simulink model "TV_2021"  (R2017b)
settings: Solver=VariableStepAuto  StartTime=0.0  StopTime=10.0  RelTol=1e-3
undefined symbols (not defined in the file): sigbuilder_block
libraries: simulink x6
(part 1 of 13)
settings Model: Creator=Eric  LastModifiedBy=GERARD
settings DataIOCC: ReturnWorkspaceOutputs=on
settings SFSimCC: SimUseLocalCustomCode=on
settings RTWCC: RTWUseLocalCustomCode=on

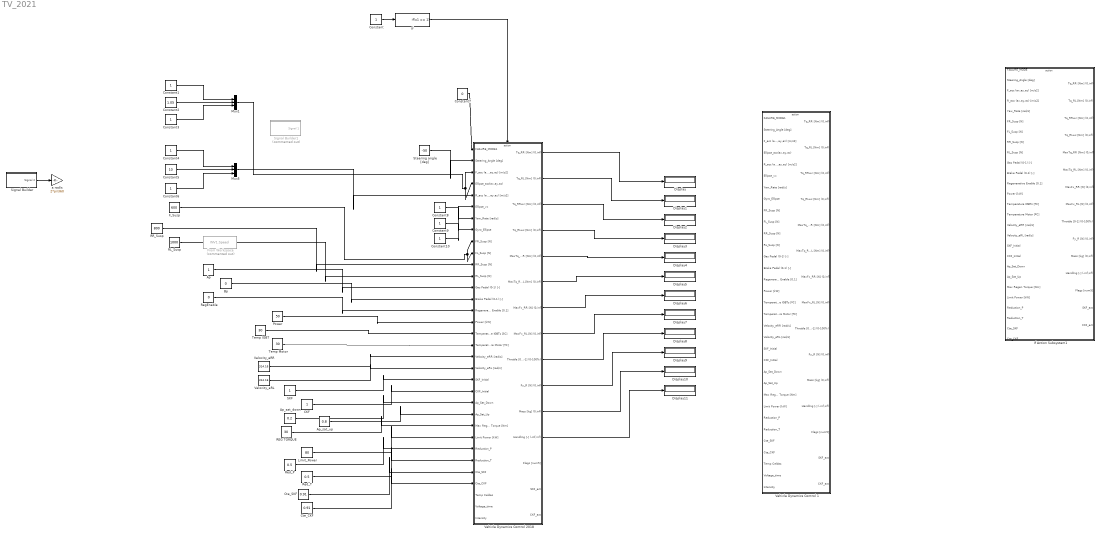
== system TV_2021 ==
  Ap : Constant
  Ap_sat_down : Constant  Value=0.2
  Ap_sat_up : Constant  Value=0.8
  Bp : Constant  Value=0
  CKF : Constant
  Constant{,1,3..4,6,8..10} (8 alike) : Constant
  Constant2 : Constant  Value=1.05
  Constant5 : Constant  Value=10
  Constant7 : Constant  Value=0
  Cte_CKF : Constant  Value=0.91
  Cte_SKF : Constant  Value=0.91
  Display{,1..11} (12 alike) : Display
  F_Susp : Constant  Value=600
  From Workspace : FromWorkspace  Commented=on  VariableName=INV1.Speed  SampleTime=0.05  OutputAfterFinalValue=Holding final value
  If : If  IfExpression=u1 == 1  ShowElse=off
  If Action Subsystem1 : Subsystem  TreatAsAtomicUnit=on
  Limit_Power : Constant  Value=80
  Mux1 : Mux  Inputs=3
  Mux5 : Mux  Inputs=3
  Power : Constant  Value=50
  REG TORQUE : Constant  Value=30
  RL_Susp : Constant  Value=1000
  RR_Susp : Constant  Value=800
  Red_P : Constant  Value=0.5
  Red_T : Constant  Value=0.5
  RegEnable : Constant  Value=0
  SKF : Constant
  Signal Builder : Subsystem  Tag=STV Subsys  LoadFcn=sigbuilder_block('load');  StartFcn=sigbuilder_block('start');  StopFcn=sigbuilder_block('stop');  ClipboardFcn=sigbuilder_block('clipboard');  mask(Sigbuilder block){tuvar=[0:10]}
      mask help: Simulink:masks:SigbuilderBlock_MD
      mask init:
      | if ~strcmp(get_param(bdroot(gcbh),'SimulationStatus'),'stopped') tuvar = sigbuilder_block('maskInit'); end
      settings: CopyFcn=sigbuilder_block('copy');  DeleteFcn=sigbuilder_block('delete');  ModelCloseFcn=sigbuilder_block('modelClose');  PreSaveFcn=sigbuilder_block('preSave');  PauseFcn=sigbuilder_block('pause');  ContinueFcn=sigbuilder_block('continue');  NameChangeFcn=sigbuilder_block('namechange');  OpenFcn=sigbuilder_block('open',[5.4 33 1141.2 514.8 ]);  CloseFcn=sigbuilder_block('close');
      mask Display: plot(0, 0, 100, 100,[2, 2, 32, 32, 2], [68, 8, 8, 68, 68],[32, 2], [38, 38], [32, 19, 2],[53, 60, 44], [32, 17, 17, 2],[16, 16, 31, 31]);txt = getActiveGroup(gcbh);text(2, 100, txt,'verticalAlignment', 'top');
  Signal Builder1 : Subsystem  Tag=STV Subsys  Commented=on  LoadFcn=sigbuilder_block('load');  StartFcn=sigbuilder_block('start');  StopFcn=sigbuilder_block('stop');  ClipboardFcn=sigbuilder_block('clipboard');  mask(Sigbuilder block){tuvar=[0:10]}
      mask help: Simulink:masks:SigbuilderBlock_MD
      mask init:
      | if ~strcmp(get_param(bdroot(gcbh),'SimulationStatus'),'stopped') tuvar = sigbuilder_block('maskInit'); end
      settings: CopyFcn=sigbuilder_block('copy');  DeleteFcn=sigbuilder_block('delete');  ModelCloseFcn=sigbuilder_block('modelClose');  PreSaveFcn=sigbuilder_block('preSave');  PauseFcn=sigbuilder_block('pause');  ContinueFcn=sigbuilder_block('continue');  NameChangeFcn=sigbuilder_block('namechange');  OpenFcn=sigbuilder_block('open',[5.4 33 1141.2 516.6 ]);  CloseFcn=sigbuilder_block('close');
      mask Display: plot(0, 0, 100, 100,[2, 2, 32, 32, 2], [68, 8, 8, 68, 68],[32, 2], [38, 38], [32, 19, 2],[53, 60, 44], [32, 17, 17, 2],[16, 16, 31, 31]);txt = getActiveGroup(gcbh);text(2, 100, txt,'verticalAlignment', 'top');
  Steering angle [deg] : Constant  Value=-50
  Temp IGBT : Constant  Value=30
  Temp Motor : Constant  Value=30
  Vehicle Dynamics Control 1 : Subsystem
  Vehicle Dynamics Control 2018 : Subsystem
  Velocity_eRL : Constant  Value=314.16
  Velocity_eRR : Constant  Value=314.16
  a rad/s : Gain  Gain=2*pi/360
  wires:
  If/1 -> Vehicle Dynamics Control 2018/Action
  Constant/1 -> If/1
  Vehicle Dynamics Control 2018/1(Tq_RR [Nm] (0,inf)) -> Display/1
  Vehicle Dynamics Control 2018/2(Tq_RL [Nm] (0,inf)) -> Display1/1
  Vehicle Dynamics Control 2018/3(Tq_RRwc [Nm] (0,inf)) -> Display2/1
  Vehicle Dynamics Control 2018/4(Tq_RLwc [Nm] (0,inf)) -> Display3/1
  Vehicle Dynamics Control 2018/5(MaxTq_RR [Nm] (0,inf)) -> Display4/1
  Vehicle Dynamics Control 2018/6(MaxTq_RL [Nm] (0,inf)) -> Display5/1
  Vehicle Dynamics Control 2018/7(MaxFx_RR [N] (0,inf)) -> Display6/1
  Vehicle Dynamics Control 2018/8(MaxFx_RL [N] (0,inf)) -> Display7/1
  Vehicle Dynamics Control 2018/9(Throttle [0-1] (0-100%)) -> Display8/1
  Vehicle Dynamics Control 2018/10(Fy_R [N] (0,inf)) -> Display9/1
  Vehicle Dynamics Control 2018/11(Mass [kg] (0,inf)) -> Display10/1
  Vehicle Dynamics Control 2018/12(Handling [-] (-inf,inf)) -> Display11/1
  Bp/1 -> Vehicle Dynamics Control 2018/14(Brake Pedal (0-1) [-])
  RegEnable/1 -> Vehicle Dynamics Control 2018/15(Regenerative Enable [0,1])
  Red_T/1 -> Vehicle Dynamics Control 2018/28(Reduction_T)
  Cte_CKF/1 -> Vehicle Dynamics Control 2018/30(Cte_CKF)
  Red_P/1 -> Vehicle Dynamics Control 2018/27(Reduction_P)
  Constant5/1 -> Mux5/2
  Constant1/1 -> Mux1/1
  Mux1/1 -> Vehicle Dynamics Control 2018/4(Ellipse_acc(ax,ay,az)), Vehicle Dynamics Control 2018/3(F_acc (ax,ay,az) [m/s2])
  Mux5/1 -> Vehicle Dynamics Control 2018/5(R_acc (ax,ay,az) [m/s2])
  Constant6/1 -> Mux5/3
  Constant3/1 -> Mux1/3
  Velocity_eRR/1 -> Vehicle Dynamics Control 2018/19(Velocity_eRR [rad/s])
  RL_Susp/1 -> Vehicle Dynamics Control 2018/12(RL_Susp [N])
  Constant4/1 -> Mux5/1
  Cte_SKF/1 -> Vehicle Dynamics Control 2018/29(Cte_SKF)
  SKF/1 -> Vehicle Dynamics Control 2018/21(SKF_Initial)
  Velocity_eRL/1 -> Vehicle Dynamics Control 2018/20(Velocity_eRL [rad/s])
  Limit_Power/1 -> Vehicle Dynamics Control 2018/26(Limit Power [kW])
  F_Susp/1 -> Vehicle Dynamics Control 2018/9(FR_Susp [N]), Vehicle Dynamics Control 2018/10(FL_Susp [N])
  Ap/1 -> Vehicle Dynamics Control 2018/13(Gas Pedal (0-1) [-])
  CKF/1 -> Vehicle Dynamics Control 2018/22(CKF_Initial)
  Signal Builder/1(Signal 2) -> a rad/s/1
  Steering angle [deg]/1 -> Vehicle Dynamics Control 2018/2(Steering_Angle [deg])
  Constant2/1 -> Mux1/2
  Constant7/1 -> Vehicle Dynamics Control 2018/1(FAILURE_MODE1)
  REG TORQUE/1 -> Vehicle Dynamics Control 2018/25(Max Regen Torque [Nm])
  Ap_sat_up/1 -> Vehicle Dynamics Control 2018/24(Ap_Sat_Up)
  Ap_sat_down/1 -> Vehicle Dynamics Control 2018/23(Ap_Sat_Down)
  Temp Motor/1 -> Vehicle Dynamics Control 2018/18(Temperature Motor [ºC])
  Temp IGBT/1 -> Vehicle Dynamics Control 2018/17(Temperature IGBTs [ºC])
  Power/1 -> Vehicle Dynamics Control 2018/16(Power [kW])
  RR_Susp/1 -> Vehicle Dynamics Control 2018/11(RR_Susp [N])
  Constant8/1 -> Vehicle Dynamics Control 2018/6(Ellipse_vx)
  Constant9/1 -> Vehicle Dynamics Control 2018/7(Yaw_Rate [rad/s])
  Constant10/1 -> Vehicle Dynamics Control 2018/8(Gyro_Ellipse)

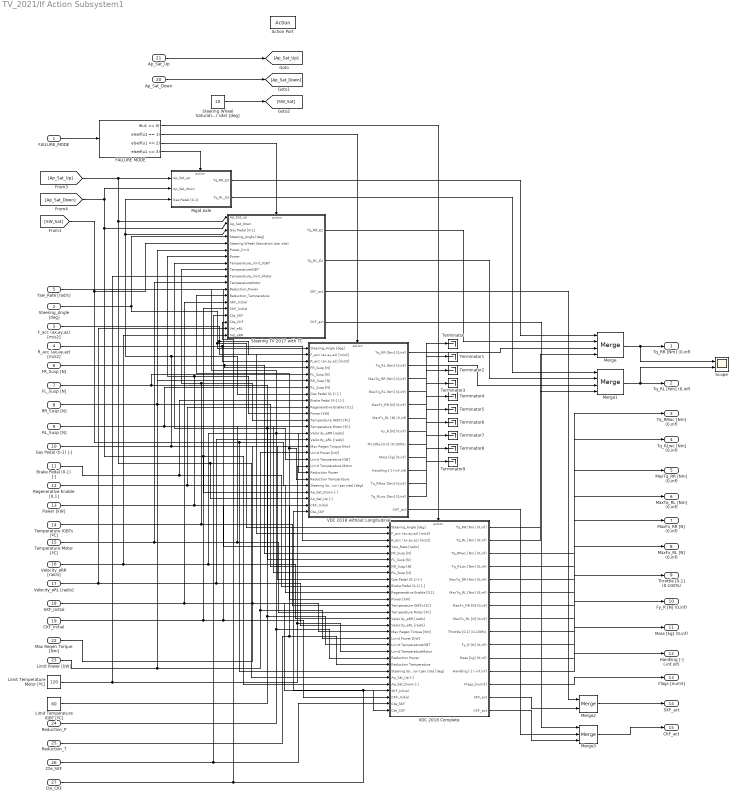
== system TV_2021/If Action Subsystem1 ==
  FAILURE_MODE : Inport
  Steering_Angle [deg] : Inport  Port=2
  F_acc (ax,ay,az) [m/s2] : Inport  Port=3
  R_acc (ax,ay,az) [m/s2] : Inport  Port=4
  Yaw_Rate [rad/s] : Inport  Port=5
  FR_Susp [N] : Inport  Port=6
  FL_Susp [N] : Inport  Port=7
  RR_Susp [N] : Inport  Port=8
  RL_Susp [N] : Inport  Port=9
  Gas Pedal (0-1) [-] : Inport  Port=10
  Brake Pedal (0-1) [-] : Inport  Port=11
  Regenerative Enable [0,1] : Inport  Port=12
  Power [kW] : Inport  Port=13
  Temperature IGBTs [ºC] : Inport  Port=14
  Temperature Motor [ºC] : Inport  Port=15
  Velocity_eRR [rad/s] : Inport  Port=16
  Velocity_eRL [rad/s] : Inport  Port=17
  SKF_Initial : Inport  Port=18
  CKF_Initial : Inport  Port=19
  Ap_Sat_Down : Inport  Port=20
  Ap_Sat_Up : Inport  Port=21
  Max Regen Torque [Nm] : Inport  Port=22
  Limit Power [kW] : Inport  Port=23
  Reduction_P : Inport  Port=24
  Reduction_T : Inport  Port=25
  Cte_SKF : Inport  Port=26
  Cte_CKF : Inport  Port=27
  Action Port : ActionPort
  FAILURE MODE : If  IfExpression=u1 == 0  ElseIfExpressions=u1 == 1, u1 == 2, u1 == 3  ShowElse=off
  Limit Temperature IGBT [ºC] : Constant  Value=60
  Limit Temperature Motor [ºC] : Constant  Value=120
  Merge : Merge  Inputs=4
  Merge1 : Merge  Inputs=4
  Merge2 : Merge
  Merge3 : Merge  Inputs=3
  Rigid Axle : Subsystem  TreatAsAtomicUnit=on
  Scope : Scope  NumInputPorts=2
  Steering TV 2017 with TC : Subsystem  TreatAsAtomicUnit=on
  "Steering Wheel Saturation (per site) [deg] " : Constant  Value=10
  Terminator{,1..9} (10 alike) : Terminator
  VDC 2018 Complete : Subsystem  TreatAsAtomicUnit=on
  VDC 2018 without Longitudinal : Subsystem  TreatAsAtomicUnit=on
  Tq_RR [Nm] (0,inf) : Outport
  Tq_RL [Nm] (0,inf) : Outport  Port=2
  Tq_RRwc [Nm] (0,inf) : Outport  Port=3
  Tq_RLwc [Nm] (0,inf) : Outport  Port=4
  MaxTq_RR [Nm] (0,inf) : Outport  Port=5
  MaxTq_RL [Nm] (0,inf) : Outport  Port=6
  MaxFx_RR [N] (0,inf) : Outport  Port=7
  MaxFx_RL [N] (0,inf) : Outport  Port=8
  Throttle [0-1] (0-100%) : Outport  Port=9
  Fy_R [N] (0,inf) : Outport  Port=10
  Mass [kg] (0,inf) : Outport  Port=11
  Handling [-] (-inf,inf) : Outport  Port=12
  Flags [num5] : Outport  Port=13
  SKF_act : Outport  Port=14
  CKF_act : Outport  Port=15
  wires:
  RL_Susp [N]/1 -> VDC 2018 Complete/8(RL_Susp [N]), VDC 2018 without Longitudinal/7(RL_Susp [N])
  R_acc (ax,ay,az) [m/s2]/1 -> VDC 2018 Complete/3(R_acc (ax,ay,az) [m/s2]), VDC 2018 without Longitudinal/3(R_acc (ax,ay,az) [m/s2])
  Steering TV 2017 with TC/4(CKF_act) -> Merge3/1
  Cte_SKF/1 -> Steering TV 2017 with TC/16(Cte_SKF), VDC 2018 Complete/28(Cte_SKF)
  VDC 2018 without Longitudinal/13(CKF_act) -> Merge3/2
  Steering TV 2017 with TC/3(SKF_act) -> Merge2/1
  Merge3/1 -> CKF_act/1
  VDC 2018 Complete/10(Fy_R [N] (0,inf)) -> Fy_R [N] (0,inf)/1
  Yaw_Rate [rad/s]/1 -> VDC 2018 Complete/4(Yaw_Rate [rad/s])
  VDC 2018 without Longitudinal/2(Tq_RL [Nm] (0,inf)) -> Merge1/3
  Merge2/1 -> SKF_act/1
  VDC 2018 Complete/15(CKF_act) -> Merge3/3
  VDC 2018 without Longitudinal/12(Tq_RLwc [Nm] (0,inf)) -> Terminator9/1
  VDC 2018 without Longitudinal/9(Mass [kg] (0,inf)) -> Terminator6/1
  Gas Pedal (0-1) [-]/1 -> VDC 2018 Complete/9(Gas Pedal (0-1) [-]), Steering TV 2017 with TC/3(Gas Pedal [0-1]), Rigid Axle/3(Gas Pedal [0-1]), VDC 2018 without Longitudinal/8(Gas Pedal (0-1) [-])
  Limit Temperature IGBT [ºC]/1 -> VDC 2018 without Longitudinal/18(Limit Temperature IGBT), Steering TV 2017 with TC/8(Temperature_limit_IGBT), VDC 2018 Complete/19(Limit TemperatureIGBT)
  SKF_Initial/1 -> VDC 2018 Complete/26(SKF_Initial), Steering TV 2017 with TC/14(SKF_Initial)
  Cte_CKF/1 -> Steering TV 2017 with TC/17(Cte_CKF), VDC 2018 without Longitudinal/26(Cte_CKF), VDC 2018 Complete/29(Cte_CKF)
  VDC 2018 Complete/13(Flags_[num5]) -> Flags [num5]/1
  VDC 2018 without Longitudinal/4(MaxTq_RL [Nm] (0,inf)) -> Terminator1/1
  VDC 2018 without Longitudinal/11(Tq_RRwc [Nm] (0,inf)) -> Terminator8/1
  Steering_Angle [deg]/1 -> VDC 2018 Complete/1(Steering_Angle [deg]), VDC 2018 without Longitudinal/1(Steering_Angle [deg]), Steering TV 2017 with TC/4(Steering_Angle [deg])
  Reduction_P/1 -> Steering TV 2017 with TC/12(Reduction_Power), VDC 2018 without Longitudinal/20(Reduction Power), VDC 2018 Complete/21(Reduction Power)
  VDC 2018 without Longitudinal/3(MaxTq_RR [Nm] (0,inf)) -> Terminator/1
  Brake Pedal (0-1) [-]/1 -> VDC 2018 Complete/10(Brake Pedal (0-1) [-]), VDC 2018 without Longitudinal/9(Brake Pedal (0-1) [-])
  VDC 2018 without Longitudinal/6(MaxFx_RL [N] (0,inf)) -> Terminator3/1
  VDC 2018 Complete/11(Mass [kg] (0,inf)) -> Mass [kg] (0,inf)/1
  Velocity_eRR [rad/s]/1 -> Steering TV 2017 with TC/19(Vel_eRR), VDC 2018 without Longitudinal/14(Velocity_eRR [rad/s]), VDC 2018 Complete/15(Velocity_eRR [rad/s])
  VDC 2018 without Longitudinal/8(Throttle [0-1] (0-100%)) -> Terminator5/1
  F_acc (ax,ay,az) [m/s2]/1 -> VDC 2018 Complete/2(F_acc (ax,ay,az) [m/s2]), VDC 2018 without Longitudinal/2(F_acc (ax,ay,az) [m/s2])
  VDC 2018 without Longitudinal/7(Fy_R [N] (0,inf)) -> Terminator4/1
  Ap_Sat_Up/1 -> [Ap_Sat_Up]
  Merge/1 -> Scope/1, Tq_RR [Nm] (0,inf)/1
  VDC 2018 Complete/12(Handling [-] (-inf,inf)) -> Handling [-] (-inf,inf)/1
  VDC 2018 without Longitudinal/1(Tq_RR [Nm] (0,inf)) -> Merge/3
  Max Regen Torque [Nm]/1 -> VDC 2018 without Longitudinal/16(Max Regen Torque [Nm]), VDC 2018 Complete/17(Max Regen Torque [Nm])
  FR_Susp [N]/1 -> VDC 2018 without Longitudinal/4(FR_Susp [N]), VDC 2018 Complete/5(FR_Susp [N])
  VDC 2018 Complete/4(Tq_RLwc [Nm] (0,inf)) -> Tq_RLwc [Nm] (0,inf)/1
  VDC 2018 without Longitudinal/5(MaxFx_RR [N] (0,inf)) -> Terminator2/1
  VDC 2018 Complete/3(Tq_RRwc [Nm] (0,inf)) -> Tq_RRwc [Nm] (0,inf)/1
  Limit Temperature Motor [ºC]/1 -> VDC 2018 without Longitudinal/19(Limit Temperature Motor), VDC 2018 Complete/20(Limit TemperatureMotor), Steering TV 2017 with TC/10(Temperature_limit_Motor)
  Rigid Axle/2(Tq_RL_E3) -> Merge1/1
  VDC 2018 Complete/9(Throttle [0-1] (0-100%)) -> Throttle [0-1] (0-100%)/1
  Reduction_T/1 -> Steering TV 2017 with TC/13(Reduction_Temperature), VDC 2018 without Longitudinal/21(Reduction Temperature), VDC 2018 Complete/22(Reduction Temperature)
  [Ap_Sat_Up] -> Rigid Axle/1("Ap_Sat_up "), VDC 2018 Complete/24(Ap_Sat_Up [-]), VDC 2018 without Longitudinal/24(Ap_Sat_Up [-]), Steering TV 2017 with TC/1("Ap_Sat_up ")
  Temperature Motor [ºC]/1 -> VDC 2018 without Longitudinal/13(Temperature Motor [ºC]), VDC 2018 Complete/14(Temperature Motor [ºC]), Steering TV 2017 with TC/11(TemperatureMotor)
  VDC 2018 Complete/6(MaxTq_RL [Nm] (0,inf)) -> MaxTq_RL [Nm] (0,inf)/1
  CKF_Initial/1 -> Steering TV 2017 with TC/15(CKF_Initial), VDC 2018 without Longitudinal/25(CKF_Initial), VDC 2018 Complete/27(CKF_Initial)
  Velocity_eRL [rad/s]/1 -> Steering TV 2017 with TC/18(Vel_eRL), VDC 2018 without Longitudinal/15(Velocity_eRL [rad/s]), VDC 2018 Complete/16(Velocity_eRL [rad/s])
  VDC 2018 Complete/7(MaxFx_RR [N] (0,inf)) -> MaxFx_RR [N] (0,inf)/1
  VDC 2018 Complete/5(MaxTq_RR [Nm] (0,inf)) -> MaxTq_RR [Nm] (0,inf)/1
  VDC 2018 Complete/1(Tq_RR [Nm] (0,inf)) -> Merge/4
  Power [kW]/1 -> Steering TV 2017 with TC/7(Power), VDC 2018 without Longitudinal/11(Power [kW]), VDC 2018 Complete/12(Power [kW])
  VDC 2018 Complete/2(Tq_RL [Nm] (0,inf)) -> Merge1/4
  RR_Susp [N]/1 -> VDC 2018 without Longitudinal/6(RR_Susp [N]), VDC 2018 Complete/7(RR_Susp [N])
  VDC 2018 without Longitudinal/10(Handling [-] (-inf,inf)) -> Terminator7/1
  [SW_Sat] -> Steering TV 2017 with TC/5("Steering Wheel Saturation (per site) "), VDC 2018 Complete/23(Steering Saturation (per site) [deg]), VDC 2018 without Longitudinal/22(Steering Saturation (per site) [deg])
  Regenerative Enable [0,1]/1 -> VDC 2018 Complete/11(Regenerative Enable [0,1]), VDC 2018 without Longitudinal/10(Regenerative Enable [0,1])
  Limit Power [kW]/1 -> Steering TV 2017 with TC/6(Power_limit), VDC 2018 without Longitudinal/17(Limit Power [kW]), VDC 2018 Complete/18(Limit Power [kW])
  FAILURE MODE/3 -> Steering TV 2017 with TC/Action
  VDC 2018 Complete/14(SKF_act) -> Merge2/2
  [Ap_Sat_Down] -> VDC 2018 Complete/25(Ap_Sat_Down [-]), VDC 2018 without Longitudinal/23(Ap_Sat_Down [-]), Steering TV 2017 with TC/2(Ap_Sat_down), Rigid Axle/2(Ap_Sat_down)
  Steering TV 2017 with TC/2(Tq_RL_E2) -> Merge1/2
  Temperature IGBTs [ºC]/1 -> VDC 2018 Complete/13(Temperature IGBTs [ºC]), Steering TV 2017 with TC/9(TemperatureIGBT), VDC 2018 without Longitudinal/12(Temperature IGBTs [ºC])
  "Steering Wheel Saturation (per site) [deg] "/1 -> [SW_Sat]
  VDC 2018 Complete/8(MaxFx_RL [N] (0,inf)) -> MaxFx_RL [N] (0,inf)/1
  FL_Susp [N]/1 -> VDC 2018 without Longitudinal/5(FL_Susp [N]), VDC 2018 Complete/6(FL_Susp [N])
  Ap_Sat_Down/1 -> [Ap_Sat_Down]
  Merge1/1 -> Scope/2, Tq_RL [Nm] (0,inf)/1
  FAILURE MODE/4 -> Rigid Axle/Action
  Rigid Axle/1(Tq_RR_E3) -> Merge/1
  Steering TV 2017 with TC/1(Tq_RR_E2) -> Merge/2
  FAILURE_MODE/1 -> FAILURE MODE/1
  FAILURE MODE/1 -> VDC 2018 Complete/Action
  FAILURE MODE/2 -> VDC 2018 without Longitudinal/Action

== system TV_2021/Signal Builder ==
  Demux : Demux  Tag=STV Demux  Outputs=1
  FromWs : FromWorkspace  Tag=STV FromWs  VariableName=tuvar  SampleTime=0
      SigBuilderData=|
      | common.afterFinalStr = 'Extrapolate'
      | common.sampleTime = 0
      | dataSet.timeRange = [0 50]
      | dataSet.name = 'Group 1'
      | sbobj.Groups.Name = 'Group 1'
      | sbobj.Groups.Signals.Name = 'Signal 2'
      | sbobj.Groups.Signals.XData = [0 50]
      | sbobj.Groups.Signals.YData = [0 -150]
      | sbobj.Groups.TimeRange = [0 50]
  Signal 2 : Outport  Tag=STV Outport
  wires:
  FromWs/1 -> Demux/1
  Demux/1 -> Signal 2/1

== system TV_2021/Signal Builder1 ==
  Demux : Demux  Tag=STV Demux  Outputs=1
  FromWs : FromWorkspace  Tag=STV FromWs  VariableName=tuvar  SampleTime=0
      SigBuilderData=|
      | common.afterFinalStr = 'Extrapolate'
      | common.sampleTime = 0
      | dataSet.timeRange = [0 50]
      | dataSet.name = 'Group 1'
      | sbobj.Groups.Name = 'Group 1'
      | sbobj.Groups.Signals.Name = 'Signal 1'
      | sbobj.Groups.Signals.XData = [0 30 30 50]
      | sbobj.Groups.Signals.YData = [20 20 30 30]
      | sbobj.Groups.TimeRange = [0 50]
  Signal 1 : Outport  Tag=STV Outport
  wires:
  FromWs/1 -> Demux/1
  Demux/1 -> Signal 1/1

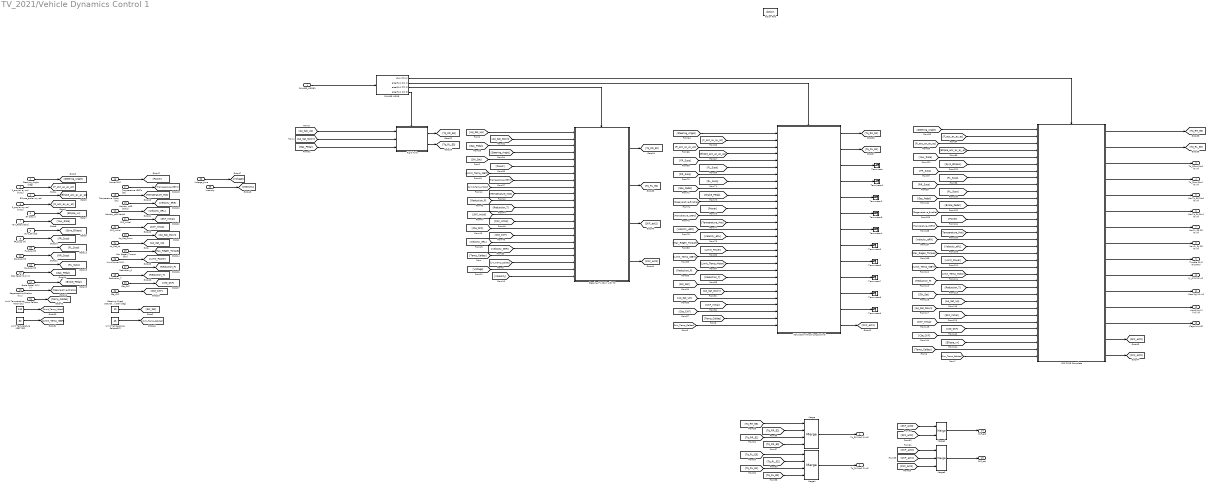
== system TV_2021/Vehicle Dynamics Control 1 ==
  FAILURE_MODE1 : Inport
  Steering_Angle [deg] : Inport  Port=2
  F_acc (ax,ay,az) [m/s2] : Inport  Port=3
  Ellipse_acc(ax,ay,az) : Inport  Port=4
  R_acc (ax,ay,az) [m/s2] : Inport  Port=5
  Ellipse_vx : Inport  Port=6
  Yaw_Rate [rad/s] : Inport  Port=7
  Gyro_Ellipse : Inport  Port=8
  FR_Susp [N] : Inport  Port=9
  FL_Susp [N] : Inport  Port=10
  RR_Susp [N] : Inport  Port=11
  RL_Susp [N] : Inport  Port=12
  Gas Pedal (0-1) [-] : Inport  Port=13
  Brake Pedal (0-1) [-] : Inport  Port=14
  Regenerative Enable [0,1] : Inport  Port=15
  Power [kW] : Inport  Port=16
  Temperature IGBTs [ºC] : Inport  Port=17
  Temperature Motor [ºC] : Inport  Port=18
  Velocity_eRR [rad/s] : Inport  Port=19
  Velocity_eRL [rad/s] : Inport  Port=20
  SKF_Initial : Inport  Port=21
  CKF_Initial : Inport  Port=22
  Ap_Sat_Down : Inport  Port=23
  Ap_Sat_Up : Inport  Port=24
  Max Regen Torque [Nm] : Inport  Port=25
  Limit Power [kW] : Inport  Port=26
  Reduction_P : Inport  Port=27
  Reduction_T : Inport  Port=28
  Cte_SKF : Inport  Port=29
  Cte_CKF : Inport  Port=30
  Temp Celdas : Inport  Port=31
  Voltage_time : Inport  Port=32
  Intensity : Inport  Port=33
  Action Port : ActionPort
  FAILURE MODE : If  IfExpression=u1 == 0  ElseIfExpressions=u1 == 1, u1 == 2, u1 == 3  ShowElse=off
  Limit Temperature Celdas[ºC] : Constant  Value=45
  Limit Temperature IGBT [ºC] : Constant  Value=60
  Limit Temperature Motor [ºC] : Constant  Value=110
  Merge : Merge  Inputs=4
  Merge1 : Merge  Inputs=4
  Merge2 : Merge
  Merge3 : Merge  Inputs=3
  Rigid Axle : Subsystem  TreatAsAtomicUnit=on
  Steering TV 2017 with TC : Subsystem  TreatAsAtomicUnit=on
  "Steering Wheel Saturation (per site) [deg] " : Constant  Value=10
  Terminator{,1..9} (10 alike) : Terminator
  VDC 2018 Complete : Subsystem  TreatAsAtomicUnit=on
  VDC 2018 without Longitudinal : Subsystem  TreatAsAtomicUnit=on
  Tq_RR [Nm] (0,inf) : Outport
  Tq_RL [Nm] (0,inf) : Outport  Port=2
  Tq_RRwc [Nm] (0,inf) : Outport  Port=3
  Tq_RLwc [Nm] (0,inf) : Outport  Port=4
  MaxTq_RR [Nm] (0,inf) : Outport  Port=5
  MaxTq_RL [Nm] (0,inf) : Outport  Port=6
  MaxFx_RR [N] (0,inf) : Outport  Port=7
  MaxFx_RL [N] (0,inf) : Outport  Port=8
  Throttle [0-1] (0-100%) : Outport  Port=9
  Fy_R [N] (0,inf) : Outport  Port=10
  Mass [kg] (0,inf) : Outport  Port=11
  Handling [-] (-inf,inf) : Outport  Port=12
  Flags [num5] : Outport  Port=13
  SKF_act : Outport  Port=14
  CKF_act : Outport  Port=15
  wires:
  [Intensity] -> Steering TV 2017 with TC/22(Corriente)
  [Voltage] -> Steering TV 2017 with TC/21(Voltage)
  Intensity/1 -> [Intensity]
  Voltage_time/1 -> [Voltage]
  [Lim_Temp_Celdas] -> VDC 2018 Complete/34(Limit_Temp_Celdas)
  [Temp_Celdas] -> VDC 2018 Complete/33(Temp_Celdas)
  [Lim_Temp_Celdas] -> VDC 2018 without Longitudinal/29(Lim_Temp_Celdas)
  [Temp_Celdas] -> VDC 2018 without Longitudinal/28(Temp_Celdas)
  [Lim_Temp_Celdas] -> Steering TV 2017 with TC/20(Lim_Temp_Celdas)
  [Temp_Celdas] -> Steering TV 2017 with TC/19(Temp_Celdas)
  Limit Temperature Celdas[ºC]/1 -> [Lim_Temp_Celdas]
  Temp Celdas/1 -> [Temp_Celdas]
  FAILURE MODE/4 -> Rigid Axle/Action
  FAILURE MODE/3 -> Steering TV 2017 with TC/Action
  FAILURE MODE/2 -> VDC 2018 without Longitudinal/Action
  FAILURE_MODE1/1 -> FAILURE MODE/1
  FAILURE MODE/1 -> VDC 2018 Complete/Action
  [Ellipse_vx] -> VDC 2018 Complete/32(Ellipse_vx)
  [SKF_Initial] -> VDC 2018 Complete/28(SKF_Initial)
  [Cte_SKF] -> VDC 2018 Complete/30(Cte_SKF)
  [Cte_CKF] -> VDC 2018 Complete/31(Cte_CKF)
  [Gyro_Ellipse] -> VDC 2018 Complete/6(Gyro_Ellipse)
  [Yaw_Rate] -> VDC 2018 Complete/5(Yaw_Rate [rad/s])
  [CKF_Initial] -> VDC 2018 Complete/29(CKF_Initial)
  [Ap_Sat_Up] -> VDC 2018 Complete/26(Ap_Sat_Up [-])
  [Ap_Sat_Down] -> VDC 2018 Complete/27(Ap_Sat_Down [-])
  [SW_Sat] -> VDC 2018 Complete/25(Steering Saturation (per site) [deg])
  [Reduction_T] -> VDC 2018 Complete/24(Reduction Temperature)
  [Reduction_P] -> VDC 2018 Complete/23(Reduction Power)
  [Limit_Temp_Motor] -> VDC 2018 Complete/22(Limit TemperatureMotor)
  [Limit_Temp_IGBT] -> VDC 2018 Complete/21(Limit TemperatureIGBT)
  [Limit_Power] -> VDC 2018 Complete/20(Limit Power [kW])
  [Max_Regen_Torque] -> VDC 2018 Complete/19(Max Regen Torque [Nm])
  [Velocity_eRL] -> VDC 2018 Complete/18(Velocity_eRL [rad/s])
  [Velocity_eRR] -> VDC 2018 Complete/17(Velocity_eRR [rad/s])
  [Temperature_Mot] -> VDC 2018 Complete/16(Temperature Motor [ºC])
  [Temperature_IGBTs] -> VDC 2018 Complete/15(Temperature IGBTs [ºC])
  [Regenerative_Enable] -> VDC 2018 Complete/13(Regenerative Enable [0,1])
  [Power] -> VDC 2018 Complete/14(Power [kW])
  [Brake_Pedal] -> VDC 2018 Complete/12(Brake Pedal (0-1) [-])
  [Gas_Pedal] -> VDC 2018 Complete/11(Gas Pedal (0-1) [-])
  [RL_Susp] -> VDC 2018 Complete/10(RL_Susp [N])
  [RR_Susp] -> VDC 2018 Complete/9(RR_Susp [N])
  [FL_Susp] -> VDC 2018 Complete/8(FL_Susp [N])
  [FR_Susp] -> VDC 2018 Complete/7(FR_Susp [N])
  [Ellipse_acc_ax_ay_az] -> VDC 2018 Complete/4(Ellipse_acc)
  [R_acc_ax_ay_az] -> VDC 2018 Complete/3(R_acc (ax,ay,az) [m/s2])
  [F_acc_ax_ay_az] -> VDC 2018 Complete/2(F_acc (ax,ay,az) [m/s2])
  [Steering_Angle] -> VDC 2018 Complete/1(Steering_Angle [deg])
  [CKF_Initial] -> VDC 2018 without Longitudinal/26(CKF_Initial)
  [SW_Sat] -> VDC 2018 without Longitudinal/23(Steering Saturation (per site) [deg])
  [Ap_Sat_Down] -> VDC 2018 without Longitudinal/24(Ap_Sat_Down [-])
  [Ap_Sat_Up] -> VDC 2018 without Longitudinal/25(Ap_Sat_Up [-])
  [Reduction_T] -> VDC 2018 without Longitudinal/22(Reduction Temperature)
  [Reduction_P] -> VDC 2018 without Longitudinal/21(Reduction Power)
  [Cte_CKF] -> VDC 2018 without Longitudinal/27(Cte_CKF)
  [Limit_Temp_Motor] -> VDC 2018 without Longitudinal/20(Limit Temperature Motor)
  [Limit_Temp_IGBT] -> VDC 2018 without Longitudinal/19(Limit Temperature IGBT)
  [Limit_Power] -> VDC 2018 without Longitudinal/18(Limit Power [kW])
  [Max_Regen_Torque] -> VDC 2018 without Longitudinal/17(Max Regen Torque [Nm])
  [Velocity_eRL] -> VDC 2018 without Longitudinal/16(Velocity_eRL [rad/s])
  [Velocity_eRR] -> VDC 2018 without Longitudinal/15(Velocity_eRR [rad/s])
  [Temperature_Mot] -> VDC 2018 without Longitudinal/14(Temperature Motor [ºC])
  [Temperature_IGBTs] -> VDC 2018 without Longitudinal/13(Temperature IGBTs [ºC])
  [Power] -> VDC 2018 without Longitudinal/12(Power [kW])
  [Regenerative_Enable] -> VDC 2018 without Longitudinal/11(Regenerative Enable [0,1])
  [Brake_Pedal] -> VDC 2018 without Longitudinal/10(Brake Pedal (0-1) [-])
  [Gas_Pedal] -> VDC 2018 without Longitudinal/9(Gas Pedal (0-1) [-])
  [RL_Susp] -> VDC 2018 without Longitudinal/8(RL_Susp [N])
  [RR_Susp] -> VDC 2018 without Longitudinal/7(RR_Susp [N])
  [FL_Susp] -> VDC 2018 without Longitudinal/6(FL_Susp [N])
  [FR_Susp] -> VDC 2018 without Longitudinal/5(FR_Susp [N])
  [R_acc_ax_ay_az] -> VDC 2018 without Longitudinal/3(R_acc (ax,ay,az) [m/s2])
  [Ellipse_acc_ax_ay_az] -> VDC 2018 without Longitudinal/4(Ellipse_acc_ax_ay_az)
  [F_acc_ax_ay_az] -> VDC 2018 without Longitudinal/2(F_acc (ax,ay,az) [m/s2])
  [Steering_Angle] -> VDC 2018 without Longitudinal/1(Steering_Angle [deg])
  [SKF_act2] -> Merge2/2
  [SKF_act0] -> Merge2/1
  [CKF_act2] -> Merge3/3
  [CKF_act0] -> Merge3/1
  [CKF_act1] -> Merge3/2
  VDC 2018 Complete/15(CKF_act) -> [CKF_act0]
  VDC 2018 Complete/14(SKF_act) -> [SKF_act0]
  VDC 2018 without Longitudinal/13(CKF_act) -> [CKF_act1]
  Steering TV 2017 with TC/4(CKF_act) -> [CKF_act2]
  Steering TV 2017 with TC/3(SKF_act) -> [SKF_act2]
  [Tq_RL_E0] -> Merge1/4
  [Tq_RR_E0] -> Merge/4
  VDC 2018 Complete/2(Tq_RL [Nm] (0,inf)) -> [Tq_RL_E0]
  VDC 2018 Complete/1(Tq_RR [Nm] (0,inf)) -> [Tq_RR_E0]
  [Tq_RL_E1] -> Merge1/3
  [Tq_RR_E1] -> Merge/3
  VDC 2018 without Longitudinal/1(Tq_RR [Nm] (0,inf)) -> [Tq_RR_E1]
  VDC 2018 without Longitudinal/2(Tq_RL [Nm] (0,inf)) -> [Tq_RL_E1]
  [Tq_RR_E2] -> Merge/2
  [Tq_RL_E2] -> Merge1/2
  Steering TV 2017 with TC/2(Tq_RL_E2) -> [Tq_RL_E2]
  Steering TV 2017 with TC/1(Tq_RR_E2) -> [Tq_RR_E2]
  [Tq_RR_E3] -> Merge/1
  [Tq_RL_E3] -> Merge1/1
  Rigid Axle/2(Tq_RL_E3) -> [Tq_RL_E3]
  Rigid Axle/1(Tq_RR_E3) -> [Tq_RR_E3]
  [Velocity_eRR] -> Steering TV 2017 with TC/18(Vel_eRR)
  [Velocity_eRL] -> Steering TV 2017 with TC/17(Vel_eRL)
  [Cte_CKF] -> Steering TV 2017 with TC/16(Cte_CKF)
  [Cte_SKF] -> Steering TV 2017 with TC/15(Cte_SKF)
  [CKF_Initial] -> Steering TV 2017 with TC/14(CKF_Initial)
  [SKF_Initial] -> Steering TV 2017 with TC/13(SKF_Initial)
  [Reduction_T] -> Steering TV 2017 with TC/12(Reduction_Temperature)
  [Reduction_P] -> Steering TV 2017 with TC/11(Reduction_Power)
  [Temperature_Mot] -> Steering TV 2017 with TC/10(TemperatureMotor)
  [Temperature_IGBTs] -> Steering TV 2017 with TC/8(TemperatureIGBT)
  [Limit_Temp_IGBT] -> Steering TV 2017 with TC/7(Temperature_limit_IGBT)
  [Limit_Temp_Motor] -> Steering TV 2017 with TC/9(Temperature_limit_Motor)
  Limit Temperature IGBT [ºC]/1 -> [Limit_Temp_IGBT]
  Limit Temperature Motor [ºC]/1 -> [Limit_Temp_Motor]
  [Power] -> Steering TV 2017 with TC/6(Power)
  [SW_Sat] -> Steering TV 2017 with TC/5("Steering Wheel Saturation (per site) ")
  [Steering_Angle] -> Steering TV 2017 with TC/4(Steering_Angle [deg])
  [Gas_Pedal] -> Steering TV 2017 with TC/3(Gas Pedal [0-1])
  [Ap_Sat_Down] -> Steering TV 2017 with TC/2(Ap_Sat_down)
  [Ap_Sat_Up] -> Steering TV 2017 with TC/1("Ap_Sat_up ")
  [Gas_Pedal] -> Rigid Axle/3(Gas Pedal [0-1])
  Cte_CKF/1 -> [Cte_CKF]
  Cte_SKF/1 -> [Cte_SKF]
  Reduction_T/1 -> [Reduction_T]
  Reduction_P/1 -> [Reduction_P]
  Limit Power [kW]/1 -> [Limit_Power]
  Max Regen Torque [Nm]/1 -> [Max_Regen_Torque]
  CKF_Initial/1 -> [CKF_Initial]
  SKF_Initial/1 -> [SKF_Initial]
  Velocity_eRL [rad/s]/1 -> [Velocity_eRL]
  Velocity_eRR [rad/s]/1 -> [Velocity_eRR]
  Temperature Motor [ºC]/1 -> [Temperature_Mot]
  Temperature IGBTs [ºC]/1 -> [Temperature_IGBTs]
  Power [kW]/1 -> [Power]
  Regenerative Enable [0,1]/1 -> [Regenerative_Enable]
  Brake Pedal (0-1) [-]/1 -> [Brake_Pedal]
  Gas Pedal (0-1) [-]/1 -> [Gas_Pedal]
  RL_Susp [N]/1 -> [RL_Susp]
  RR_Susp [N]/1 -> [RR_Susp]
  FL_Susp [N]/1 -> [FL_Susp]
  FR_Susp [N]/1 -> [FR_Susp]
  Gyro_Ellipse/1 -> [Gyro_Ellipse]
  Yaw_Rate [rad/s]/1 -> [Yaw_Rate]
  Ellipse_vx/1 -> [Ellipse_vx]
  R_acc (ax,ay,az) [m/s2]/1 -> [R_acc_ax_ay_az]
  Ellipse_acc(ax,ay,az)/1 -> [Ellipse_acc_ax_ay_az]
  F_acc (ax,ay,az) [m/s2]/1 -> [F_acc_ax_ay_az]
  Steering_Angle [deg]/1 -> [Steering_Angle]
  Merge3/1 -> CKF_act/1
  Merge2/1 -> SKF_act/1
  VDC 2018 Complete/13(Flags_[num5]) -> Flags [num5]/1
  Ap_Sat_Up/1 -> [Ap_Sat_Up]
  VDC 2018 without Longitudinal/12(Tq_RLwc [Nm] (0,inf)) -> Terminator9/1
  VDC 2018 without Longitudinal/11(Tq_RRwc [Nm] (0,inf)) -> Terminator8/1
  VDC 2018 without Longitudinal/10(Handling [-] (-inf,inf)) -> Terminator7/1
  VDC 2018 without Longitudinal/9(Mass [kg] (0,inf)) -> Terminator6/1
  VDC 2018 without Longitudinal/8(Throttle [0-1] (0-100%)) -> Terminator5/1
  VDC 2018 without Longitudinal/7(Fy_R [N] (0,inf)) -> Terminator4/1
  VDC 2018 without Longitudinal/6(MaxFx_RL [N] (0,inf)) -> Terminator3/1
  VDC 2018 without Longitudinal/5(MaxFx_RR [N] (0,inf)) -> Terminator2/1
  VDC 2018 without Longitudinal/4(MaxTq_RL [Nm] (0,inf)) -> Terminator1/1
  VDC 2018 without Longitudinal/3(MaxTq_RR [Nm] (0,inf)) -> Terminator/1
  VDC 2018 Complete/12(Handling [-] (-inf,inf)) -> Handling [-] (-inf,inf)/1
  VDC 2018 Complete/11(Mass [kg] (0,inf)) -> Mass [kg] (0,inf)/1
  VDC 2018 Complete/10(Fy_R [N] (0,inf)) -> Fy_R [N] (0,inf)/1
  VDC 2018 Complete/9(Throttle [0-1] (0-100%)) -> Throttle [0-1] (0-100%)/1
  VDC 2018 Complete/8(MaxFx_RL [N] (0,inf)) -> MaxFx_RL [N] (0,inf)/1
  VDC 2018 Complete/7(MaxFx_RR [N] (0,inf)) -> MaxFx_RR [N] (0,inf)/1
  VDC 2018 Complete/6(MaxTq_RL [Nm] (0,inf)) -> MaxTq_RL [Nm] (0,inf)/1
  VDC 2018 Complete/5(MaxTq_RR [Nm] (0,inf)) -> MaxTq_RR [Nm] (0,inf)/1
  VDC 2018 Complete/3(Tq_RRwc [Nm] (0,inf)) -> Tq_RRwc [Nm] (0,inf)/1
  VDC 2018 Complete/4(Tq_RLwc [Nm] (0,inf)) -> Tq_RLwc [Nm] (0,inf)/1
  [Ap_Sat_Down] -> Rigid Axle/2(Ap_Sat_down)
  [Ap_Sat_Up] -> Rigid Axle/1("Ap_Sat_up ")
  "Steering Wheel Saturation (per site) [deg] "/1 -> [SW_Sat]
  Ap_Sat_Down/1 -> [Ap_Sat_Down]
  Merge/1 -> Tq_RR [Nm] (0,inf)/1
  Merge1/1 -> Tq_RL [Nm] (0,inf)/1

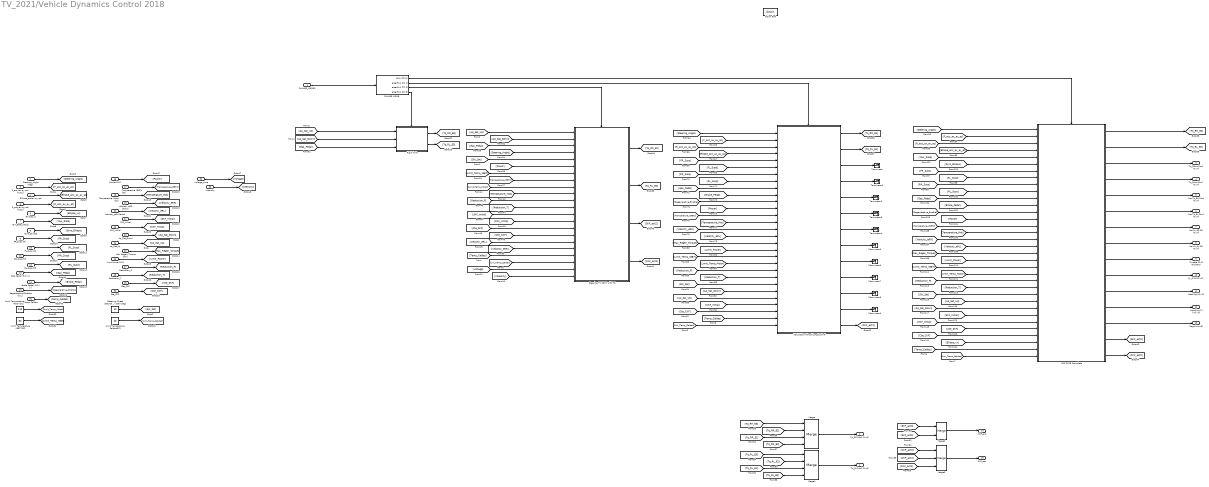
== system TV_2021/Vehicle Dynamics Control 2018 ==
  FAILURE_MODE1 : Inport
  Steering_Angle [deg] : Inport  Port=2
  F_acc (ax,ay,az) [m/s2] : Inport  Port=3
  Ellipse_acc(ax,ay,az) : Inport  Port=4
  R_acc (ax,ay,az) [m/s2] : Inport  Port=5
  Ellipse_vx : Inport  Port=6
  Yaw_Rate [rad/s] : Inport  Port=7
  Gyro_Ellipse : Inport  Port=8
  FR_Susp [N] : Inport  Port=9
  FL_Susp [N] : Inport  Port=10
  RR_Susp [N] : Inport  Port=11
  RL_Susp [N] : Inport  Port=12
  Gas Pedal (0-1) [-] : Inport  Port=13
  Brake Pedal (0-1) [-] : Inport  Port=14
  Regenerative Enable [0,1] : Inport  Port=15
  Power [kW] : Inport  Port=16
  Temperature IGBTs [ºC] : Inport  Port=17
  Temperature Motor [ºC] : Inport  Port=18
  Velocity_eRR [rad/s] : Inport  Port=19
  Velocity_eRL [rad/s] : Inport  Port=20
  SKF_Initial : Inport  Port=21
  CKF_Initial : Inport  Port=22
  Ap_Sat_Down : Inport  Port=23
  Ap_Sat_Up : Inport  Port=24
  Max Regen Torque [Nm] : Inport  Port=25
  Limit Power [kW] : Inport  Port=26
  Reduction_P : Inport  Port=27
  Reduction_T : Inport  Port=28
  Cte_SKF : Inport  Port=29
  Cte_CKF : Inport  Port=30
  Temp Celdas : Inport  Port=31
  Voltage_time : Inport  Port=32
  Intensity : Inport  Port=33
  Action Port : ActionPort
  FAILURE MODE : If  IfExpression=u1 == 0  ElseIfExpressions=u1 == 1, u1 == 2, u1 == 3  ShowElse=off
  Limit Temperature Celdas[ºC] : Constant  Value=45
  Limit Temperature IGBT [ºC] : Constant  Value=60
  Limit Temperature Motor [ºC] : Constant  Value=110
  Merge : Merge  Inputs=4
  Merge1 : Merge  Inputs=4
  Merge2 : Merge
  Merge3 : Merge  Inputs=3
  Rigid Axle : Subsystem  TreatAsAtomicUnit=on
  Steering TV 2017 with TC : Subsystem  TreatAsAtomicUnit=on
  "Steering Wheel Saturation (per site) [deg] " : Constant  Value=10
  Terminator{,1..9} (10 alike) : Terminator
  VDC 2018 Complete : Subsystem  TreatAsAtomicUnit=on
  VDC 2018 without Longitudinal : Subsystem  TreatAsAtomicUnit=on
  Tq_RR [Nm] (0,inf) : Outport
  Tq_RL [Nm] (0,inf) : Outport  Port=2
  Tq_RRwc [Nm] (0,inf) : Outport  Port=3
  Tq_RLwc [Nm] (0,inf) : Outport  Port=4
  MaxTq_RR [Nm] (0,inf) : Outport  Port=5
  MaxTq_RL [Nm] (0,inf) : Outport  Port=6
  MaxFx_RR [N] (0,inf) : Outport  Port=7
  MaxFx_RL [N] (0,inf) : Outport  Port=8
  Throttle [0-1] (0-100%) : Outport  Port=9
  Fy_R [N] (0,inf) : Outport  Port=10
  Mass [kg] (0,inf) : Outport  Port=11
  Handling [-] (-inf,inf) : Outport  Port=12
  Flags [num5] : Outport  Port=13
  SKF_act : Outport  Port=14
  CKF_act : Outport  Port=15
  wires:
  Merge1/1 -> Tq_RL [Nm] (0,inf)/1
  Merge/1 -> Tq_RR [Nm] (0,inf)/1
  Ap_Sat_Down/1 -> [Ap_Sat_Down]
  "Steering Wheel Saturation (per site) [deg] "/1 -> [SW_Sat]
  [Ap_Sat_Up] -> Rigid Axle/1("Ap_Sat_up ")
  [Ap_Sat_Down] -> Rigid Axle/2(Ap_Sat_down)
  VDC 2018 Complete/4(Tq_RLwc [Nm] (0,inf)) -> Tq_RLwc [Nm] (0,inf)/1
  VDC 2018 Complete/3(Tq_RRwc [Nm] (0,inf)) -> Tq_RRwc [Nm] (0,inf)/1
  VDC 2018 Complete/5(MaxTq_RR [Nm] (0,inf)) -> MaxTq_RR [Nm] (0,inf)/1
  VDC 2018 Complete/6(MaxTq_RL [Nm] (0,inf)) -> MaxTq_RL [Nm] (0,inf)/1
  VDC 2018 Complete/7(MaxFx_RR [N] (0,inf)) -> MaxFx_RR [N] (0,inf)/1
  VDC 2018 Complete/8(MaxFx_RL [N] (0,inf)) -> MaxFx_RL [N] (0,inf)/1
  VDC 2018 Complete/9(Throttle [0-1] (0-100%)) -> Throttle [0-1] (0-100%)/1
  VDC 2018 Complete/10(Fy_R [N] (0,inf)) -> Fy_R [N] (0,inf)/1
  VDC 2018 Complete/11(Mass [kg] (0,inf)) -> Mass [kg] (0,inf)/1
  VDC 2018 Complete/12(Handling [-] (-inf,inf)) -> Handling [-] (-inf,inf)/1
  VDC 2018 without Longitudinal/3(MaxTq_RR [Nm] (0,inf)) -> Terminator/1
  VDC 2018 without Longitudinal/4(MaxTq_RL [Nm] (0,inf)) -> Terminator1/1
  VDC 2018 without Longitudinal/5(MaxFx_RR [N] (0,inf)) -> Terminator2/1
  VDC 2018 without Longitudinal/6(MaxFx_RL [N] (0,inf)) -> Terminator3/1
  VDC 2018 without Longitudinal/7(Fy_R [N] (0,inf)) -> Terminator4/1
  VDC 2018 without Longitudinal/8(Throttle [0-1] (0-100%)) -> Terminator5/1
  VDC 2018 without Longitudinal/9(Mass [kg] (0,inf)) -> Terminator6/1
  VDC 2018 without Longitudinal/10(Handling [-] (-inf,inf)) -> Terminator7/1
  VDC 2018 without Longitudinal/11(Tq_RRwc [Nm] (0,inf)) -> Terminator8/1
  VDC 2018 without Longitudinal/12(Tq_RLwc [Nm] (0,inf)) -> Terminator9/1
  Ap_Sat_Up/1 -> [Ap_Sat_Up]
  VDC 2018 Complete/13(Flags_[num5]) -> Flags [num5]/1
  Merge2/1 -> SKF_act/1
  Merge3/1 -> CKF_act/1
  Steering_Angle [deg]/1 -> [Steering_Angle]
  F_acc (ax,ay,az) [m/s2]/1 -> [F_acc_ax_ay_az]
  Ellipse_acc(ax,ay,az)/1 -> [Ellipse_acc_ax_ay_az]
  R_acc (ax,ay,az) [m/s2]/1 -> [R_acc_ax_ay_az]
  Ellipse_vx/1 -> [Ellipse_vx]
  Yaw_Rate [rad/s]/1 -> [Yaw_Rate]
  Gyro_Ellipse/1 -> [Gyro_Ellipse]
  FR_Susp [N]/1 -> [FR_Susp]
  FL_Susp [N]/1 -> [FL_Susp]
  RR_Susp [N]/1 -> [RR_Susp]
  RL_Susp [N]/1 -> [RL_Susp]
  Gas Pedal (0-1) [-]/1 -> [Gas_Pedal]
  Brake Pedal (0-1) [-]/1 -> [Brake_Pedal]
  Regenerative Enable [0,1]/1 -> [Regenerative_Enable]
  Power [kW]/1 -> [Power]
  Temperature IGBTs [ºC]/1 -> [Temperature_IGBTs]
  Temperature Motor [ºC]/1 -> [Temperature_Mot]
  Velocity_eRR [rad/s]/1 -> [Velocity_eRR]
  Velocity_eRL [rad/s]/1 -> [Velocity_eRL]
  SKF_Initial/1 -> [SKF_Initial]
  CKF_Initial/1 -> [CKF_Initial]
  Max Regen Torque [Nm]/1 -> [Max_Regen_Torque]
  Limit Power [kW]/1 -> [Limit_Power]
  Reduction_P/1 -> [Reduction_P]
  Reduction_T/1 -> [Reduction_T]
  Cte_SKF/1 -> [Cte_SKF]
  Cte_CKF/1 -> [Cte_CKF]
  [Gas_Pedal] -> Rigid Axle/3(Gas Pedal [0-1])
  [Ap_Sat_Up] -> Steering TV 2017 with TC/1("Ap_Sat_up ")
  [Ap_Sat_Down] -> Steering TV 2017 with TC/2(Ap_Sat_down)
  [Gas_Pedal] -> Steering TV 2017 with TC/3(Gas Pedal [0-1])
  [Steering_Angle] -> Steering TV 2017 with TC/4(Steering_Angle [deg])
  [SW_Sat] -> Steering TV 2017 with TC/5("Steering Wheel Saturation (per site) ")
  [Power] -> Steering TV 2017 with TC/6(Power)
  Limit Temperature Motor [ºC]/1 -> [Limit_Temp_Motor]
  Limit Temperature IGBT [ºC]/1 -> [Limit_Temp_IGBT]
  [Limit_Temp_Motor] -> Steering TV 2017 with TC/9(Temperature_limit_Motor)
  [Limit_Temp_IGBT] -> Steering TV 2017 with TC/7(Temperature_limit_IGBT)
  [Temperature_IGBTs] -> Steering TV 2017 with TC/8(TemperatureIGBT)
  [Temperature_Mot] -> Steering TV 2017 with TC/10(TemperatureMotor)
  [Reduction_P] -> Steering TV 2017 with TC/11(Reduction_Power)
  [Reduction_T] -> Steering TV 2017 with TC/12(Reduction_Temperature)
  [SKF_Initial] -> Steering TV 2017 with TC/13(SKF_Initial)
  [CKF_Initial] -> Steering TV 2017 with TC/14(CKF_Initial)
  [Cte_SKF] -> Steering TV 2017 with TC/15(Cte_SKF)
  [Cte_CKF] -> Steering TV 2017 with TC/16(Cte_CKF)
  [Velocity_eRL] -> Steering TV 2017 with TC/17(Vel_eRL)
  [Velocity_eRR] -> Steering TV 2017 with TC/18(Vel_eRR)
  Rigid Axle/1(Tq_RR_E3) -> [Tq_RR_E3]
  Rigid Axle/2(Tq_RL_E3) -> [Tq_RL_E3]
  [Tq_RL_E3] -> Merge1/1
  [Tq_RR_E3] -> Merge/1
  Steering TV 2017 with TC/1(Tq_RR_E2) -> [Tq_RR_E2]
  Steering TV 2017 with TC/2(Tq_RL_E2) -> [Tq_RL_E2]
  [Tq_RL_E2] -> Merge1/2
  [Tq_RR_E2] -> Merge/2
  VDC 2018 without Longitudinal/2(Tq_RL [Nm] (0,inf)) -> [Tq_RL_E1]
  VDC 2018 without Longitudinal/1(Tq_RR [Nm] (0,inf)) -> [Tq_RR_E1]
  [Tq_RR_E1] -> Merge/3
  [Tq_RL_E1] -> Merge1/3
  VDC 2018 Complete/1(Tq_RR [Nm] (0,inf)) -> [Tq_RR_E0]
  VDC 2018 Complete/2(Tq_RL [Nm] (0,inf)) -> [Tq_RL_E0]
  [Tq_RR_E0] -> Merge/4
  [Tq_RL_E0] -> Merge1/4
  Steering TV 2017 with TC/3(SKF_act) -> [SKF_act2]
  Steering TV 2017 with TC/4(CKF_act) -> [CKF_act2]
  VDC 2018 without Longitudinal/13(CKF_act) -> [CKF_act1]
  VDC 2018 Complete/14(SKF_act) -> [SKF_act0]
  VDC 2018 Complete/15(CKF_act) -> [CKF_act0]
  [CKF_act1] -> Merge3/2
  [CKF_act0] -> Merge3/1
  [CKF_act2] -> Merge3/3
  [SKF_act0] -> Merge2/1
  [SKF_act2] -> Merge2/2
  [Steering_Angle] -> VDC 2018 without Longitudinal/1(Steering_Angle [deg])
  [F_acc_ax_ay_az] -> VDC 2018 without Longitudinal/2(F_acc (ax,ay,az) [m/s2])
  [Ellipse_acc_ax_ay_az] -> VDC 2018 without Longitudinal/4(Ellipse_acc_ax_ay_az)
  [R_acc_ax_ay_az] -> VDC 2018 without Longitudinal/3(R_acc (ax,ay,az) [m/s2])
  [FR_Susp] -> VDC 2018 without Longitudinal/5(FR_Susp [N])
  [FL_Susp] -> VDC 2018 without Longitudinal/6(FL_Susp [N])
  [RR_Susp] -> VDC 2018 without Longitudinal/7(RR_Susp [N])
  [RL_Susp] -> VDC 2018 without Longitudinal/8(RL_Susp [N])
  [Gas_Pedal] -> VDC 2018 without Longitudinal/9(Gas Pedal (0-1) [-])
  [Brake_Pedal] -> VDC 2018 without Longitudinal/10(Brake Pedal (0-1) [-])
  [Regenerative_Enable] -> VDC 2018 without Longitudinal/11(Regenerative Enable [0,1])
  [Power] -> VDC 2018 without Longitudinal/12(Power [kW])
  [Temperature_IGBTs] -> VDC 2018 without Longitudinal/13(Temperature IGBTs [ºC])
  [Temperature_Mot] -> VDC 2018 without Longitudinal/14(Temperature Motor [ºC])
  [Velocity_eRR] -> VDC 2018 without Longitudinal/15(Velocity_eRR [rad/s])
  [Velocity_eRL] -> VDC 2018 without Longitudinal/16(Velocity_eRL [rad/s])
  [Max_Regen_Torque] -> VDC 2018 without Longitudinal/17(Max Regen Torque [Nm])
  [Limit_Power] -> VDC 2018 without Longitudinal/18(Limit Power [kW])
  [Limit_Temp_IGBT] -> VDC 2018 without Longitudinal/19(Limit Temperature IGBT)
  [Limit_Temp_Motor] -> VDC 2018 without Longitudinal/20(Limit Temperature Motor)
  [Cte_CKF] -> VDC 2018 without Longitudinal/27(Cte_CKF)
  [Reduction_P] -> VDC 2018 without Longitudinal/21(Reduction Power)
  [Reduction_T] -> VDC 2018 without Longitudinal/22(Reduction Temperature)
  [Ap_Sat_Up] -> VDC 2018 without Longitudinal/25(Ap_Sat_Up [-])
  [Ap_Sat_Down] -> VDC 2018 without Longitudinal/24(Ap_Sat_Down [-])
  [SW_Sat] -> VDC 2018 without Longitudinal/23(Steering Saturation (per site) [deg])
  [CKF_Initial] -> VDC 2018 without Longitudinal/26(CKF_Initial)
  [Steering_Angle] -> VDC 2018 Complete/1(Steering_Angle [deg])
  [F_acc_ax_ay_az] -> VDC 2018 Complete/2(F_acc (ax,ay,az) [m/s2])
  [R_acc_ax_ay_az] -> VDC 2018 Complete/3(R_acc (ax,ay,az) [m/s2])
  [Ellipse_acc_ax_ay_az] -> VDC 2018 Complete/4(Ellipse_acc)
  [FR_Susp] -> VDC 2018 Complete/7(FR_Susp [N])
  [FL_Susp] -> VDC 2018 Complete/8(FL_Susp [N])
  [RR_Susp] -> VDC 2018 Complete/9(RR_Susp [N])
  [RL_Susp] -> VDC 2018 Complete/10(RL_Susp [N])
  [Gas_Pedal] -> VDC 2018 Complete/11(Gas Pedal (0-1) [-])
  [Brake_Pedal] -> VDC 2018 Complete/12(Brake Pedal (0-1) [-])
  [Power] -> VDC 2018 Complete/14(Power [kW])
  [Regenerative_Enable] -> VDC 2018 Complete/13(Regenerative Enable [0,1])
  [Temperature_IGBTs] -> VDC 2018 Complete/15(Temperature IGBTs [ºC])
  [Temperature_Mot] -> VDC 2018 Complete/16(Temperature Motor [ºC])
  [Velocity_eRR] -> VDC 2018 Complete/17(Velocity_eRR [rad/s])
  [Velocity_eRL] -> VDC 2018 Complete/18(Velocity_eRL [rad/s])
  [Max_Regen_Torque] -> VDC 2018 Complete/19(Max Regen Torque [Nm])
  [Limit_Power] -> VDC 2018 Complete/20(Limit Power [kW])
  [Limit_Temp_IGBT] -> VDC 2018 Complete/21(Limit TemperatureIGBT)
  [Limit_Temp_Motor] -> VDC 2018 Complete/22(Limit TemperatureMotor)
  [Reduction_P] -> VDC 2018 Complete/23(Reduction Power)
  [Reduction_T] -> VDC 2018 Complete/24(Reduction Temperature)
  [SW_Sat] -> VDC 2018 Complete/25(Steering Saturation (per site) [deg])
  [Ap_Sat_Down] -> VDC 2018 Complete/27(Ap_Sat_Down [-])
  [Ap_Sat_Up] -> VDC 2018 Complete/26(Ap_Sat_Up [-])
  [CKF_Initial] -> VDC 2018 Complete/29(CKF_Initial)
  [Yaw_Rate] -> VDC 2018 Complete/5(Yaw_Rate [rad/s])
  [Gyro_Ellipse] -> VDC 2018 Complete/6(Gyro_Ellipse)
  [Cte_CKF] -> VDC 2018 Complete/31(Cte_CKF)
  [Cte_SKF] -> VDC 2018 Complete/30(Cte_SKF)
  [SKF_Initial] -> VDC 2018 Complete/28(SKF_Initial)
  [Ellipse_vx] -> VDC 2018 Complete/32(Ellipse_vx)
  FAILURE MODE/1 -> VDC 2018 Complete/Action
  FAILURE_MODE1/1 -> FAILURE MODE/1
  FAILURE MODE/2 -> VDC 2018 without Longitudinal/Action
  FAILURE MODE/3 -> Steering TV 2017 with TC/Action
  FAILURE MODE/4 -> Rigid Axle/Action
  Temp Celdas/1 -> [Temp_Celdas]
  Limit Temperature Celdas[ºC]/1 -> [Lim_Temp_Celdas]
  [Temp_Celdas] -> Steering TV 2017 with TC/19(Temp_Celdas)
  [Lim_Temp_Celdas] -> Steering TV 2017 with TC/20(Lim_Temp_Celdas)
  [Temp_Celdas] -> VDC 2018 without Longitudinal/28(Temp_Celdas)
  [Lim_Temp_Celdas] -> VDC 2018 without Longitudinal/29(Lim_Temp_Celdas)
  [Temp_Celdas] -> VDC 2018 Complete/33(Temp_Celdas)
  [Lim_Temp_Celdas] -> VDC 2018 Complete/34(Limit_Temp_Celdas)
  Voltage_time/1 -> [Voltage]
  Intensity/1 -> [Intensity]
  [Voltage] -> Steering TV 2017 with TC/21(Voltage)
  [Intensity] -> Steering TV 2017 with TC/22(Corriente)

== system TV_2021/If Action Subsystem1/Rigid Axle ==
  "Ap_Sat_up " : Inport
  Ap_Sat_down : Inport  Port=2
  Gas Pedal [0-1] : Inport  Port=3
  Action Port : ActionPort
  Accelerating : Subsystem
  Torque_RL [Nm] : Constant  Value=60
  Torque_RR [Nm] : Constant  Value=60
  Tq_RR_E3 : Outport
  Tq_RL_E3 : Outport  Port=2
  wires:
  Gas Pedal [0-1]/1 -> Accelerating/1(Ap)
  "Ap_Sat_up "/1 -> Accelerating/2("Ap_Sat_up ")
  Ap_Sat_down/1 -> Accelerating/3(Ap_Sat_down)
  Accelerating/1("Tq_RR ") -> Tq_RR_E3/1
  Accelerating/2(Tq_RL) -> Tq_RL_E3/1
  Torque_RR [Nm]/1 -> Accelerating/4(Tq_RR)
  Torque_RL [Nm]/1 -> Accelerating/5("Tq_RL ")

== system TV_2021/If Action Subsystem1/Steering TV 2017 with TC ==
  "Ap_Sat_up " : Inport
  Ap_Sat_down : Inport  Port=2
  Gas Pedal [0-1] : Inport  Port=3
  Steering_Angle [deg] : Inport  Port=4
  "Steering Wheel Saturation (per site) " : Inport  Port=5
  Power_limit : Inport  Port=6
  Power : Inport  Port=7
  Temperature_limit_IGBT : Inport  Port=8
  TemperatureIGBT : Inport  Port=9
  Temperature_limit_Motor : Inport  Port=10
  TemperatureMotor : Inport  Port=11
  Reduction_Power : Inport  Port=12
  Reduction_Temperature : Inport  Port=13
  SKF_Initial : Inport  Port=14
  CKF_Initial : Inport  Port=15
  Cte_SKF : Inport  Port=16
  Cte_CKF : Inport  Port=17
  Vel_eRL : Inport  Port=18
  Vel_eRR : Inport  Port=19
  Action Port : ActionPort
  Accelerating : Subsystem
  Constraints : Subsystem
  Display : Display
  Display1 : Display
  If : If  NumInputs=2  IfExpression=-u2 <= u1 & u1 <= u2
  Lateral Dynamics : Subsystem  TreatAsAtomicUnit=on
  Longitudinal Dynamics : Subsystem  TreatAsAtomicUnit=on
  MATLAB Function1 : MATLAB Function  TreatAsAtomicUnit=on
  Merge : Merge
  Merge1 : Merge
  Mux : Mux  Inputs=2
  Optimization SKF & CKF : Subsystem
  Scope : Scope
  Scope1 : Scope  NumInputPorts=2
  Steering TV 2017 without TC : MATLAB Function  TreatAsAtomicUnit=on
  Steering Wheel Maximum Angle : Constant  Value=140
  Tq_diff_max [Nm] : Constant  Value=100
  Tq_max [Nm] : Constant  Value=130
  Tq_RR_E2 : Outport
  Tq_RL_E2 : Outport  Port=2
  SKF_act : Outport  Port=3
  CKF_act : Outport  Port=4
  wires:
  Gas Pedal [0-1]/1 -> Accelerating/1(Ap)
  "Ap_Sat_up "/1 -> Accelerating/2("Ap_Sat_up ")
  Ap_Sat_down/1 -> Accelerating/3(Ap_Sat_down)
  Tq_max [Nm]/1 -> Steering TV 2017 without TC/4(tq_max)
  Tq_diff_max [Nm]/1 -> Steering TV 2017 without TC/5(tq_max_diff)
  Steering Wheel Maximum Angle/1 -> Steering TV 2017 without TC/3(sw_max_angle), MATLAB Function1/1(cte)
  "Steering Wheel Saturation (per site) "/1 -> If/2, Steering TV 2017 without TC/2(sw_saturation)
  Steering TV 2017 without TC/1(tq_RR) -> Lateral Dynamics/1(Tq_RR), Longitudinal Dynamics/1(Tq_RR)
  Steering TV 2017 without TC/2(tq_RL) -> Lateral Dynamics/2(Tq_RL), Longitudinal Dynamics/2(Tq_RL)
  Power_limit/1 -> Constraints/1(Power_limit)
  Power/1 -> Constraints/2(Power)
  Temperature_limit_IGBT/1 -> Constraints/3(Temperature_limit_IGBT)
  TemperatureIGBT/1 -> Constraints/4(Temperature_IGBT)
  Reduction_Temperature/1 -> Constraints/9(ReductionCte_Temperature)
  Reduction_Power/1 -> Constraints/10(ReductionCte_Power)
  Constraints/1(TQ_RR) -> Scope1/1, Tq_RR_E2/1
  Constraints/2(TQ_RL) -> Scope1/2, Tq_RL_E2/1
  Accelerating/2(Tq_RL) -> Constraints/8(Tq_RL)
  Accelerating/1("Tq_RR ") -> Constraints/7(Tq_RR)
  MATLAB Function1/1(value) -> Steering TV 2017 without TC/1(sw_angle), If/1
  Temperature_limit_Motor/1 -> Constraints/5(Temperature_limit_Motor)
  TemperatureMotor/1 -> Constraints/6(Temperature_Motor)
  Optimization SKF & CKF/2(CKF_act) -> Display1/1, Mux/1, Lateral Dynamics/3(CKF), CKF_act/1
  SKF_Initial/1 -> Optimization SKF & CKF/4(SKF_Initial)
  Mux/1 -> Scope/1
  Cte_SKF/1 -> Optimization SKF & CKF/6(Cte_SKF)
  Vel_eRL/1 -> Optimization SKF & CKF/1(RPM_INV1)
  Vel_eRR/1 -> Optimization SKF & CKF/2(RPM_INV2)
  Optimization SKF & CKF/1(SKF_act) -> SKF_act/1, Longitudinal Dynamics/3(SKF), Display/1, Mux/2
  Steering_Angle [deg]/1 -> MATLAB Function1/2(v), Optimization SKF & CKF/3(Steer_An)
  CKF_Initial/1 -> Optimization SKF & CKF/5(CKF_Initial)
  Cte_CKF/1 -> Optimization SKF & CKF/7(Cte_CKF)
  If/1 -> Longitudinal Dynamics/Action
  Lateral Dynamics/2(Tq_RL_with_CKF) -> Merge1/2
  If/2 -> Lateral Dynamics/Action
  Longitudinal Dynamics/2(Tq_RL_with_SKF) -> Merge1/1
  Longitudinal Dynamics/1(Tq_RR_with_SKF) -> Merge/1
  Lateral Dynamics/1(Tq_RR_with_CKF) -> Merge/2
  Merge/1 -> Accelerating/4(Tq_RR)
  Merge1/1 -> Accelerating/5("Tq_RL ")
